simulink library "csc_imu_sensor_prep_lib"  (R2014b)
settings: Solver=ode45  SolverMode=SingleTasking  StartTime=0.0  StopTime=10.0  RelTol=1e-3
values from neighbouring files (symbols this model uses):
  stg_body_to_head1_dcm = [ 0.0000    1.0000         0 ... (first row only)    [csc_stg_tracker_sensor_prep_init.m]
  stg_miru_gyro_to_body_dcm = [ 0.0000   -1.0000         0 ... (first row only)    [csc_stg_tracker_sensor_prep_init.m]
undefined symbols (not defined in the file or in its folder): kfl_use_mems, mum1_dcm
libraries: util_info_lib x1
settings Model: ExtModeAutoUpdateStatusClock=off  Creator=Administrator  LastModifiedBy=Mark Wells

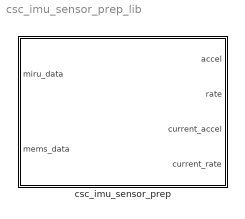
== system csc_imu_sensor_prep_lib ==
  csc_imu_sensor_prep : Subsystem

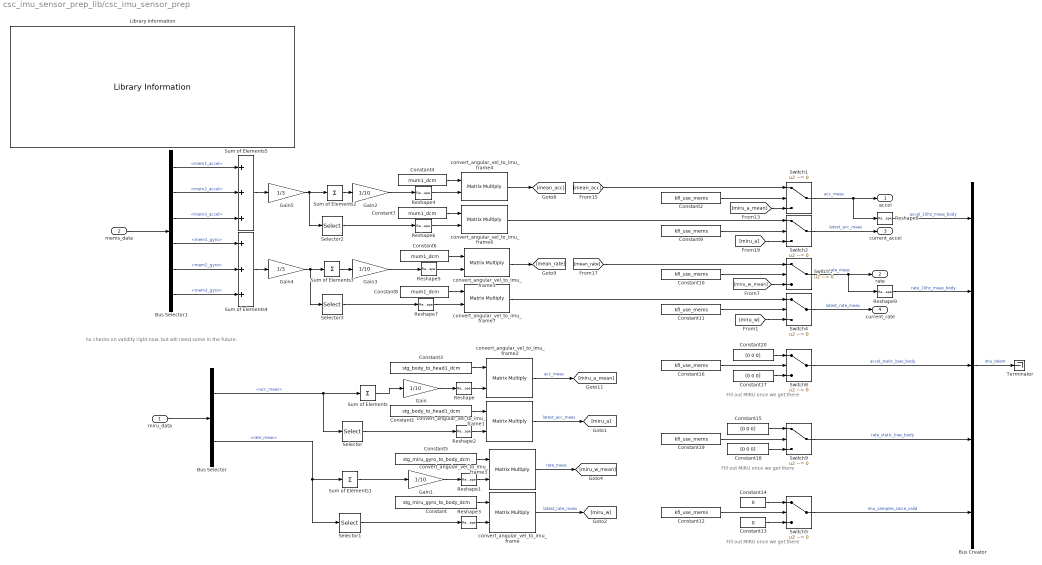
== system csc_imu_sensor_prep_lib/csc_imu_sensor_prep ==
  note: Fill out MIRU once we get there
  note: Fill out MIRU once we get there
  note: no checks on validity right now, but will need some in the future.
  note: Fill out MIRU once we get there
  miru_data : Inport
  mems_data : Inport  Port=2
  Bus Creator : BusCreator  Inputs=5
  Bus Selector : BusSelector  OutputSignals=acc_meas,rate_meas
  Bus Selector1 : BusSelector  OutputSignals=mem1_accel,mem2_accel,mem3_accel,mem1_gyro,mem2_gyro,mem3_gyro
  Constant : Constant  Value=stg_miru_gyro_to_body_dcm
  Constant1 : Constant  Value=stg_body_to_head1_dcm
  Constant{2,9..12,16,19} (7 alike) : Constant  Value=kfl_use_mems
  Constant13 : Constant  Value=0  OutDataTypeStr=uint8
  Constant14 : Constant  Value=0  OutDataTypeStr=uint8
  Constant{15,17..18,20} (4 alike) : Constant  Value=[0 0 0]  OutDataTypeStr=double
  Constant3 : Constant  Value=stg_body_to_head1_dcm
  Constant{4,6..8} (4 alike) : Constant  Value=mum1_dcm
  Constant5 : Constant  Value=stg_miru_gyro_to_body_dcm
  Gain{,1..3} (4 alike) : Gain  Gain=1/10
  Gain4 : Gain  Gain=1/3
  Gain5 : Gain  Gain=1/3
  Library Information : util_info_lib/Library Information  owner='escrane'
  Reshape{,1..7} (8 alike) : Reshape  OutputDimensionality=Column vector (2-D)
  Reshape8 : Reshape
  Reshape9 : Reshape
  Selector{,1..3} (4 alike) : Selector  NumberOfDimensions=2  InputPortWidth=3  IndexOptions=Index vector (dialog),Select all  Indices=1,1  OutputSizes=1,1
  Sum of Elements{,1..3} (4 alike) : Sum  Inputs=+  CollapseMode=Specified dimension
  Sum of Elements4 : Sum  Inputs=+++  CollapseMode=Specified dimension
  Sum of Elements5 : Sum  Inputs=+++  CollapseMode=Specified dimension
  Switch{1..5,8..9} (7 alike) : Switch  Criteria=u2 ~= 0
  Terminator : Terminator
  convert_angular_vel_to_imu_frame{,1..7} (8 alike) : Product  Multiplication=Matrix(*)  RndMeth=Zero
  accel : Outport
  rate : Outport  Port=2
  current_accel : Outport  Port=3
  current_rate : Outport  Port=4
  wires:
  [mean_rate] -> Switch3/1
  [mean_acc] -> Switch1/1
  convert_angular_vel_to_imu_frame6/1 -> Switch2/1
  Selector2/1 -> Reshape6/1
  convert_angular_vel_to_imu_frame5/1 -> [mean_rate]
  convert_angular_vel_to_imu_frame4/1 -> [mean_acc]
  convert_angular_vel_to_imu_frame7/1 -> Switch4/1
  Gain3/1 -> Reshape5/1
  Gain2/1 -> Reshape4/1
  Selector3/1 -> Reshape7/1
  Bus Selector1/6 -> Sum of Elements4/3  "<mem3_gyro>"
  Bus Selector1/5 -> Sum of Elements4/2  "<mem2_gyro>"
  Switch9/1 -> Bus Creator/4  "rate_static_bias_body"
  Constant18/1 -> Switch9/3
  Constant19/1 -> Switch9/2
  Constant15/1 -> Switch9/1
  Switch8/1 -> Bus Creator/3  "accel_static_bias_body"
  Constant17/1 -> Switch8/3
  Constant16/1 -> Switch8/2
  Constant20/1 -> Switch8/1
  Reshape9/1 -> Bus Creator/2  "rate_10hz_meas_body"
  Reshape8/1 -> Bus Creator/1  "accel_10hz_meas_body"
  Switch5/1 -> Bus Creator/5  "imu_samples_since_valid"
  Constant13/1 -> Switch5/3
  Constant12/1 -> Switch5/2
  Constant14/1 -> Switch5/1
  Bus Creator/1 -> Terminator/1  "imu_telem"
  Switch4/1 -> current_rate/1  "latest_rate_meas"
  Switch3/1 -> rate/1, Reshape9/1  "rate_meas"
  [miru_w] -> Switch4/3
  [miru_w_mean] -> Switch3/3
  Constant11/1 -> Switch4/2
  Constant10/1 -> Switch3/2
  Switch2/1 -> current_accel/1  "latest_acc_meas"
  convert_angular_vel_to_imu_frame1/1 -> [miru_a]  "latest_acc_meas"
  [miru_a] -> Switch2/3
  [miru_a_mean] -> Switch1/3
  convert_angular_vel_to_imu_frame2/1 -> [miru_a_mean]  "acc_meas"
  Constant9/1 -> Switch2/2
  Switch1/1 -> accel/1, Reshape8/1  "acc_meas"
  Constant2/1 -> Switch1/2
  Constant8/1 -> convert_angular_vel_to_imu_frame7/1
  Reshape7/1 -> convert_angular_vel_to_imu_frame7/2
  Constant6/1 -> convert_angular_vel_to_imu_frame5/1
  Constant7/1 -> convert_angular_vel_to_imu_frame6/1
  Reshape6/1 -> convert_angular_vel_to_imu_frame6/2
  Constant4/1 -> convert_angular_vel_to_imu_frame4/1
  Sum of Elements4/1 -> Gain4/1
  Gain4/1 -> Sum of Elements3/1, Selector3/1
  Reshape5/1 -> convert_angular_vel_to_imu_frame5/2
  Sum of Elements3/1 -> Gain3/1
  Sum of Elements5/1 -> Gain5/1
  Gain5/1 -> Sum of Elements2/1, Selector2/1
  Bus Selector1/4 -> Sum of Elements4/1  "<mem1_gyro>"
  Reshape4/1 -> convert_angular_vel_to_imu_frame4/2
  Bus Selector1/3 -> Sum of Elements5/3  "<mem3_accel>"
  Bus Selector1/2 -> Sum of Elements5/2  "<mem2_accel>"
  Sum of Elements2/1 -> Gain2/1
  Bus Selector1/1 -> Sum of Elements5/1  "<mem1_accel>"
  mems_data/1 -> Bus Selector1/1
  Reshape3/1 -> convert_angular_vel_to_imu_frame/2
  Selector/1 -> Reshape2/1
  Reshape2/1 -> convert_angular_vel_to_imu_frame1/2
  Reshape1/1 -> convert_angular_vel_to_imu_frame3/2
  Reshape/1 -> convert_angular_vel_to_imu_frame2/2
  Sum of Elements1/1 -> Gain1/1
  Sum of Elements/1 -> Gain/1
  Constant5/1 -> convert_angular_vel_to_imu_frame3/1
  Gain1/1 -> Reshape1/1
  Bus Selector/2 -> Sum of Elements1/1, Selector1/1  "<rate_meas>"
  Gain/1 -> Reshape/1
  Constant3/1 -> convert_angular_vel_to_imu_frame2/1
  convert_angular_vel_to_imu_frame/1 -> [miru_w]  "latest_rate_meas"
  Selector1/1 -> Reshape3/1
  Constant1/1 -> convert_angular_vel_to_imu_frame1/1
  convert_angular_vel_to_imu_frame3/1 -> [miru_w_mean]  "rate_meas"
  Constant/1 -> convert_angular_vel_to_imu_frame/1
  Bus Selector/1 -> Sum of Elements/1, Selector/1  "<acc_meas>"
  miru_data/1 -> Bus Selector/1
